simulink model "CMOS_Kernel_Memory_Sync"  (R2023b)
settings: Solver=VariableStepAuto  StartTime=0.0  StopTime=30000000  RelTol=1e-3
values from neighbouring files (symbols this model uses):
  AmountOfPixelsPerScanline = 400    [Kernel_Setup_Script.m]
  AmountOfRamBlocksScanlines = 5    [Kernel_Setup_Script.m]
  AmountOfRamBlocksScanlinesOffset = AmountOfRamBlocksScanlines - 1    (= 4)    [Kernel_Setup_Script.m]
  AmountOfScanlinePixels = 73700    [Kernel_Setup_Script.m]
  AmountOfScanlinePixelsOffset = AmountOfScanlinePixels - 1    (= 73699)    [Kernel_Setup_Script.m]
  AmountOfScanlines = 1100    [Kernel_Setup_Script.m]
  AmountOfScanlinesOffset = AmountOfScanlines - 1    (= 1099)    [Kernel_Setup_Script.m]
  AOPPK_Off = AmountOfPixelsPerScanline - 1    (= 399)    [Kernel_Setup_Script.m]
  AOPPS_Off = AmountOfPixelsPerScanline - 1    (= 399)    [Kernel_Setup_Script.m]
  FramePackOff_0 = FramePackOff_0 - ScanlineFifoCheck    [Kernel_Setup_Script.m]
  FramePackOff_1 = FramePackOff_1 - ScanlineFifoCheck    [Kernel_Setup_Script.m]
  FramePackOff_2 = FramePackOff_2 - ScanlineFifoCheck    [Kernel_Setup_Script.m]
  FramePackOff_3 = FramePackOff_3 - ScanlineFifoCheck    [Kernel_Setup_Script.m]
  FramePackOff_4 = FramePackOff_4 - ScanlineFifoCheck    [Kernel_Setup_Script.m]
  FramePackOff_5 = FramePackOff_5 - ScanlineFifoCheck    [Kernel_Setup_Script.m]
  KernelPackOff_0 = KernelPackOff_0 - KernelBitsPerRow    [Kernel_Setup_Script.m]
  KernelPackOff_1 = KernelPackOff_1 - KernelBitsPerRow    [Kernel_Setup_Script.m]
  KernelPackOff_2 = KernelPackOff_2 - KernelBitsPerRow    [Kernel_Setup_Script.m]
  KernelPackOff_3 = KernelPackOff_3 - KernelBitsPerRow    [Kernel_Setup_Script.m]
  Slice59DownTo48Top = (MsbOffset - (ScanlinePixelBitSizeController*1))    (= 59)    [Kernel_Setup_Script.m]
  Slice71DownTo60Top = (MsbOffset - (ScanlinePixelBitSizeController*0))    (= 71)    [Kernel_Setup_Script.m]
  TotalSectionsForFrames = AmountOfScanlines/AmountOfRamBlocksScanlines    (= 220)    [Kernel_Setup_Script.m]
  UltraRamRows = AmountOfPixelsPerScanline/ScanlineFifoCheck    [Kernel_Setup_Script.m]
  UltraRamRowsCeil = ceil(AmountOfPixelsPerScanline/ScanlineFifoCheck)    [Kernel_Setup_Script.m]
  UltraRamRowsKernel = AmountOfPixelsPerScanline/KernelBitsPerRow    (= 100)    [Kernel_Setup_Script.m]
  UltraRamRowsKernelCeil = ceil(AmountOfPixelsPerScanline/KernelBitsPerRow)    [Kernel_Setup_Script.m]
  UltraRamRowsMemorySectionOffset = UltraRamRowsCeil*AmountOfRamBlocksScanlines    [Kernel_Setup_Script.m]
  UltraRamRowsOffset = UltraRamRowsCeil - 1    [Kernel_Setup_Script.m]
undefined symbols (not defined in the file or in its folder): c, Down, sfvc784, Up, xck26
libraries: hdlBasic x4512, vmcUtilities x1
(part 1 of 39)
settings Model: Creator=Backm  LastModifiedBy=Backm

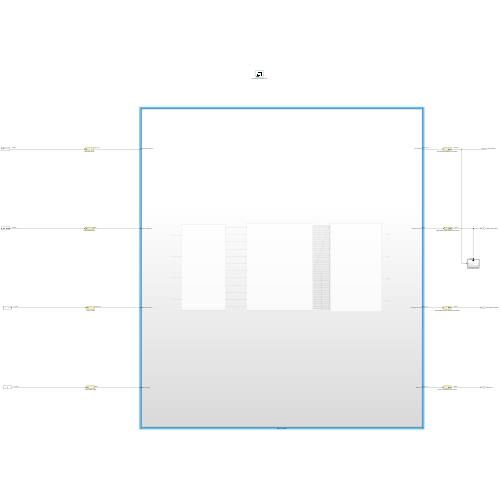
[thumbnail: Simulink's stored preview of the top-level diagram]
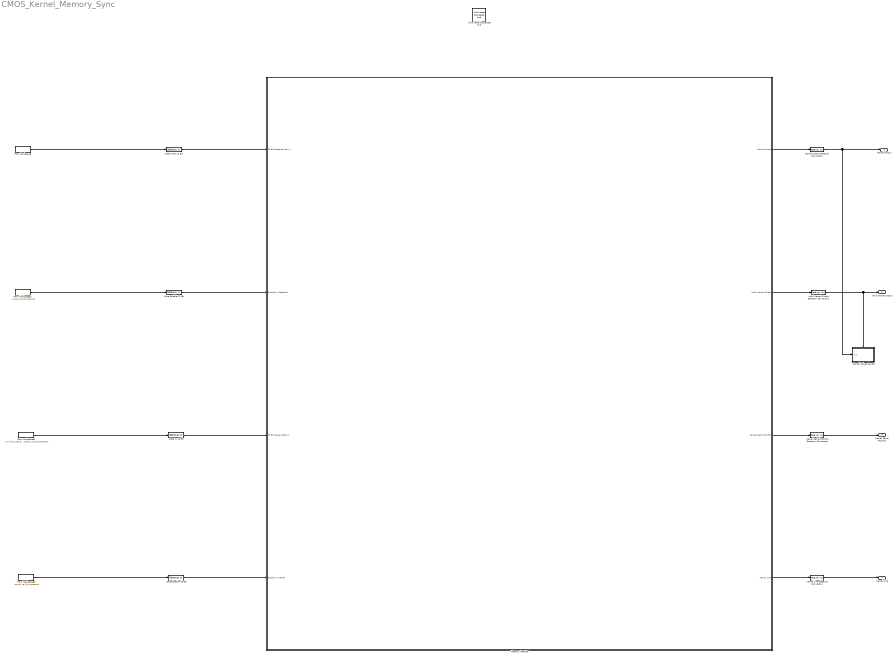
== system CMOS_Kernel_Memory_Sync ==
  Data Enable 18 Bit : hdlBasic/Gateway In  gui_display_data_type=Boolean  arith_type=Boolean  n_bits=18  bin_pt=0  preci_type=Single  exp_width=8  frac_width=24  rows=1  columns=1  quantization="Round  (unbiased: +/- Inf)"  overflow=Saturate  period=1  UseAsADC=off  ADCChannel='1'  interface=None  automatic_assignment=off  address_offset=hex2dec('00')  intf_name=''  intf_description=''  default_value=0  timing_constraint=None  locs_specified=off  LOCs={}  io_standard={}  inherit_from_input=off  hdl_port=on  XmcBlockStatus=1  maskContainerNames=group4  block_type=gatewayin  block_config=sysgen:gateway_in_config  block_width_w=590  block_height_w=620  block_width=640  block_height=850
  Data In 18 Bit : hdlBasic/Gateway In  gui_display_data_type=Fixed-point  arith_type=Unsigned  n_bits=18  bin_pt=0  preci_type=Single  exp_width=8  frac_width=24  rows=1  columns=1  quantization="Round  (unbiased: +/- Inf)"  overflow=Saturate  period=1  UseAsADC=off  ADCChannel='1'  interface=None  automatic_assignment=off  address_offset=hex2dec('00')  intf_name=''  intf_description=''  default_value=0  timing_constraint=None  locs_specified=off  LOCs={}  io_standard={}  inherit_from_input=off  hdl_port=on  XmcBlockStatus=1  maskContainerNames=group4  block_type=gatewayin  block_config=sysgen:gateway_in_config  block_width_w=590  block_height_w=620  block_width=640  block_height=850
  Data Input 12 Bit : hdlBasic/Gateway In  gui_display_data_type=Fixed-point  arith_type=Unsigned  n_bits=12  bin_pt=0  preci_type=Single  exp_width=8  frac_width=24  rows=1  columns=1  quantization="Round  (unbiased: +/- Inf)"  overflow=Saturate  period=1  UseAsADC=off  ADCChannel='1'  interface=None  automatic_assignment=off  address_offset=hex2dec('00')  intf_name=''  intf_description=''  default_value=0  timing_constraint=None  locs_specified=off  LOCs={}  io_standard={}  inherit_from_input=off  hdl_port=on  XmcBlockStatus=1  maskContainerNames=group4  block_type=gatewayin  block_config=sysgen:gateway_in_config  block_width_w=590  block_height_w=620  block_width=640  block_height=850
  From Workspace : FromWorkspace  VariableName=input_timeseries  Interpolate=off  OutputAfterFinalValue=Setting to zero
  From Workspace1 : FromWorkspace  VariableName=input_valid_timeseries  Interpolate=off  OutputAfterFinalValue=Setting to zero
  From Workspace2 : FromWorkspace  VariableName=auxillary_kernel_match_input_timeseries  Interpolate=off  OutputAfterFinalValue=Setting to zero
  From Workspace3 : FromWorkspace  VariableName=kernel_valid_timeseries  Interpolate=off  OutputAfterFinalValue=Setting to zero
  Kernel Line Gateway Conversion : hdlBasic/Gateway Out  inherit_from_input=off  hdl_port=on  rows=1  columns=1  UseAsDAC=off  DACChannel='1'  interface=None  automatic_assignment=on  address_offset=hex2dec('00')  intf_name=''  intf_description=''  timing_constraint=None  locs_specified=off  LOCs={}  io_standard={}  XmcBlockStatus=1  maskContainerNames=group4  block_type=gatewayout  block_config=sysgen:gateway_out_config  block_width_w=590  block_height_w=620  block_width=620  block_height=750
  Kernel Output Gateway Conversion : hdlBasic/Gateway Out  inherit_from_input=off  hdl_port=on  rows=1  columns=1  UseAsDAC=off  DACChannel='1'  interface=None  automatic_assignment=on  address_offset=hex2dec('00')  intf_name=''  intf_description=''  timing_constraint=None  locs_specified=off  LOCs={}  io_standard={}  XmcBlockStatus=1  maskContainerNames=group4  block_type=gatewayout  block_config=sysgen:gateway_out_config  block_width_w=590  block_height_w=620  block_width=620  block_height=750
  Kernel Serial Position Gateway Conversion : hdlBasic/Gateway Out  inherit_from_input=off  hdl_port=on  rows=1  columns=1  UseAsDAC=off  DACChannel='1'  interface=None  automatic_assignment=on  address_offset=hex2dec('00')  intf_name=''  intf_description=''  timing_constraint=None  locs_specified=off  LOCs={}  io_standard={}  XmcBlockStatus=1  maskContainerNames=group4  block_type=gatewayout  block_config=sysgen:gateway_out_config  block_width_w=590  block_height_w=620  block_width=620  block_height=750
  Kernel Values Saved : Subsystem
  Memory Handler : Subsystem
      settings: RTWMemSecFuncInitTerm=Inherit fRAM model  RTWMemSecFuncExecute=Inherit fRAM model  RTWMemSecDataConstants=Inherit fRAM model  RTWMemSecDataInternal=Inherit fRAM model  RTWMemSecDataParameters=Inherit fRAM model
  Valid Kernel Output Gateway Conversion : hdlBasic/Gateway Out  inherit_from_input=off  hdl_port=on  rows=1  columns=1  UseAsDAC=off  DACChannel='1'  interface=None  automatic_assignment=on  address_offset=hex2dec('00')  intf_name=''  intf_description=''  timing_constraint=None  locs_specified=off  LOCs={}  io_standard={}  XmcBlockStatus=1  maskContainerNames=group4  block_type=gatewayout  block_config=sysgen:gateway_out_config  block_width_w=590  block_height_w=620  block_width=620  block_height=750
  Vitis Model Composer Hub : vmcUtilities/Vitis Model Composer Hub  Tag=genX  CodeGeneration=off  SubsystemName=Frame Memory Controller  CompilationType=HDLCompilation  ExportTypeV2=IP Catalog  TargetDirectory=./netlist  exportDesign=off  analyzeDesign=off  validateDesignOnHw=off  ExportType=AI Engines  IpVendor=xilinx.com  IpLibrary=hls  IpVersion=1.0  IpHWLanguage=Verilog  AieCompilerOptions={}  AieSimulatorOptions={}  CreateTestbench=off  TestbenchStackSize=10  RunRtlSim=off  RunCSim=off  RunAieSim=off  AieSimTimeout=50000  RunAieSimProfiling=off  LaunchVitisAnalyzer=off  PlotOutput=off  RunX86Sim=off  X86SimTimeout=10  GenHwImage=off  GenLibadfXo=on  GenHwValidationCode=off  PlatformType=Not Specified  HwSystemType=Baremetal  HwValidationTarget=hw  ProjDevice=Kria KR260 Robotics Starter Kit SOM (xck26-sfvc784-2LV-c)  ProjDevicePart=xck26-sfvc784-2LV-c  SamplePeriod=-1  ClockFrequency=200  DataPathParallelism=1  xilinxfamily=zynquplus  part=xck26  speed=-2LV-c  package=sfvc784  directory=./netlist\ip\Frame_Memory_Controller\src  testbench=off  incr_netlist=off  synthesis_tool=Vivado  clock_wrapper=Clock Enables  dbl_ovrd=According to Block Masks  dcm_input_clock_period=10  sysclk_period=10  simulink_period=1/6  eval_field=0  LogFileName=''  NThreads=4
  Write Enable 12 Bit : hdlBasic/Gateway In  gui_display_data_type=Boolean  arith_type=Boolean  n_bits=16  bin_pt=14  preci_type=Single  exp_width=8  frac_width=24  rows=1  columns=1  quantization="Round  (unbiased: +/- Inf)"  overflow=Saturate  period=1  UseAsADC=off  ADCChannel='1'  interface=None  automatic_assignment=on  address_offset=hex2dec('00')  intf_name=''  intf_description=''  default_value=0  timing_constraint=None  locs_specified=off  LOCs={}  io_standard={}  inherit_from_input=off  hdl_port=on  XmcBlockStatus=1  maskContainerNames=group4  block_type=gatewayin  block_config=sysgen:gateway_in_config  block_width_w=590  block_height_w=620  block_width=640  block_height=850
  Kernel Output : Outport
  Valid Kernel Output : Outport  Port=2
  Kernel Serial Position : Outport  Port=3
  Kernel Line : Outport  Port=4
  wires:
  Kernel Line Gateway Conversion/1 -> Kernel Line/1
  Memory Handler/4(Kernel Line) -> Kernel Line Gateway Conversion/1
  Memory Handler/3(Kernel Serial Position) -> Kernel Serial Position Gateway Conversion/1
  Kernel Serial Position Gateway Conversion/1 -> Kernel Serial Position/1
  Memory Handler/2(Valid Kernel Output) -> Valid Kernel Output Gateway Conversion/1
  Valid Kernel Output Gateway Conversion/1 -> Valid Kernel Output/1, Kernel Values Saved/Enable
  Memory Handler/1(Kernel Output) -> Kernel Output Gateway Conversion/1
  Kernel Output Gateway Conversion/1 -> Kernel Output/1, Kernel Values Saved/1(In1)
  From Workspace/1 -> Data Input 12 Bit/1
  From Workspace1/1 -> Write Enable 12 Bit/1
  From Workspace2/1 -> Data In 18 Bit/1
  Data Enable 18 Bit/1 -> Memory Handler/4(Enable In Kernel)
  Data In 18 Bit/1 -> Memory Handler/3(18 Bit Kernel Data In)
  Write Enable 12 Bit/1 -> Memory Handler/2(Enable In Spectrual)
  Data Input 12 Bit/1 -> Memory Handler/1(12 Bit Spectrual Bin In)
  From Workspace3/1 -> Data Enable 18 Bit/1

== system CMOS_Kernel_Memory_Sync/Kernel Values Saved ==
  In1 : Inport
  Enable : EnablePort
  To Workspace : ToWorkspace  VariableName=simout_kernel_values_out  SampleTime=-1
      settings: Save2DSignal=2-D array (concatenate along first dimension)
  wires:
  In1/1 -> To Workspace/1

== system CMOS_Kernel_Memory_Sync/Memory Handler ==
  12 Bit Spectrual Bin In : Inport
  Enable In Spectrual : Inport  Port=2
  18 Bit Kernel Data In : Inport  Port=3
  Enable In Kernel : Inport  Port=4
  Data Slicer : Subsystem
      settings: RTWMemSecFuncInitTerm=Inherit fRAM model  RTWMemSecFuncExecute=Inherit fRAM model  RTWMemSecDataConstants=Inherit fRAM model  RTWMemSecDataInternal=Inherit fRAM model  RTWMemSecDataParameters=Inherit fRAM model
  Math : Subsystem
  Memory Manager : Subsystem
      settings: RTWMemSecFuncInitTerm=Inherit fRAM model  RTWMemSecFuncExecute=Inherit fRAM model  RTWMemSecDataConstants=Inherit fRAM model  RTWMemSecDataInternal=Inherit fRAM model  RTWMemSecDataParameters=Inherit fRAM model
  Kernel Output : Outport
  Valid Kernel Output : Outport  Port=2
  Kernel Serial Position : Outport  Port=3
  Kernel Line : Outport  Port=4
  wires:
  Memory Manager/11(Kernel RAM 4 Out1) -> Data Slicer/11(Kernel Data In RAM 4)
  12 Bit Spectrual Bin In/1 -> Memory Manager/1(12 Bit Spectrual Bin In)
  Memory Manager/2(Spectrual RAM 1 Out) -> Data Slicer/2(Data In RAM 1)
  Memory Manager/6(Spectrual Valid) -> Data Slicer/6(Frame Valid In)
  Memory Manager/4(Spectrual RAM 3 Out) -> Data Slicer/4(Data In RAM 3)
  Memory Manager/10(Kernel RAM 3 Out1) -> Data Slicer/10(Kernel Data In RAM 3)
  Memory Manager/3(Spectrual RAM 2 Out) -> Data Slicer/3(Data In RAM 2)
  Memory Manager/8(Kernel RAM 1 Out1) -> Data Slicer/8(Kernel Data In RAM 1)
  Memory Manager/9(Kernel RAM 2 Out1) -> Data Slicer/9(Kernel Data In RAM 2)
  Memory Manager/1(Spectrual RAM 0 Out) -> Data Slicer/1(Data In RAM 0)
  Memory Manager/7(Kernel RAM 0 Out1) -> Data Slicer/7(Kernel Data In RAM 0)
  Enable In Spectrual/1 -> Memory Manager/2(Enable In Spectrual)
  Memory Manager/12(" Kernel Valid") -> Data Slicer/12(Kernel Valid In)
  Memory Manager/5(Spectrual RAM 4 Out) -> Data Slicer/5(Data In RAM 4)
  Enable In Kernel/1 -> Memory Manager/4(Enable In Kernel)
  18 Bit Kernel Data In/1 -> Memory Manager/3(18 Bit Kernel Data In)
  Data Slicer/1(Frame Pixel 0 at Offset 0) -> Math/1(In Pixel 0 at Offset 0)
  Data Slicer/2(Frame Pixel 1 at Offset 0) -> Math/2(In Pixel 1 at Offset 0)
  Data Slicer/3(Frame Pixel 2 at Offset 0) -> Math/3(In Pixel 2 at Offset 0)
  Data Slicer/4(Frame Pixel 3 at Offset 0) -> Math/4(In Pixel 3 at Offset 0)
  Data Slicer/5(Frame Pixel 4 at Offset 0) -> Math/5(In Pixel 4 at Offset 0)
  Data Slicer/6(Frame Pixel 5 at Offset 0) -> Math/6(In Pixel 5 at Offset 0)
  Data Slicer/7(Frame Pixel 6 at Offset 0) -> Math/7(In Pixel 6 at Offset 0)
  Data Slicer/8(Frame Pixel 7 at Offset 0) -> Math/8(In Pixel 7 at Offset 0)
  Data Slicer/9(Frame Pixel 8 at Offset 0) -> Math/9(In Pixel 8 at Offset 0)
  Data Slicer/10(Frame Pixel 9 at Offset 0) -> Math/10(In Pixel 9 at Offset 0)
  Data Slicer/11(Frame Pixel 10 at Offset 0) -> Math/11(In Pixel 10 at Offset 0)
  Data Slicer/12(Frame Pixel 11 at Offset 0) -> Math/12(In Pixel 11 at Offset 0)
  Data Slicer/13(Frame Pixel 0 at Offset 1) -> Math/13(In Pixel 0 at Offset 1)
  Data Slicer/14(Frame Pixel 1 at Offset 1) -> Math/14(In Pixel 1 at Offset 1)
  Data Slicer/15(Frame Pixel 2 at Offset 1) -> Math/15(In Pixel 2 at Offset 1)
  Data Slicer/16(Frame Pixel 3 at Offset 1) -> Math/16(In Pixel 3 at Offset 1)
  Data Slicer/17(Frame Pixel 4 at Offset 1) -> Math/17(In Pixel 4 at Offset 1)
  Data Slicer/18(Frame Pixel 5 at Offset 1) -> Math/18(In Pixel 5 at Offset 1)
  Data Slicer/20(Frame Pixel 7 at Offset 1) -> Math/20(In Pixel 7 at Offset 1)
  Data Slicer/19(Frame Pixel 6 at Offset 1) -> Math/19(In Pixel 6 at Offset 1)
  Data Slicer/21(Frame Pixel 8 at Offset 1) -> Math/21(In Pixel 8 at Offset 1)
  Data Slicer/22(Frame Pixel 9 at Offset 1) -> Math/22(In Pixel 9 at Offset 1)
  Data Slicer/23(Frame Pixel 10 at Offset 1) -> Math/23(In Pixel 10 at Offset 1)
  Data Slicer/24(Frame Pixel 11 at Offset 1) -> Math/24(In Pixel 11 at Offset 1)
  Data Slicer/25(Frame Pixel 0 at Offset 2) -> Math/25(In Pixel 0 at Offset 2)
  Data Slicer/26(Frame Pixel 1 at Offset 2) -> Math/26(In Pixel 1 at Offset 2)
  Data Slicer/27(Frame Pixel 2 at Offset 2) -> Math/27(In Pixel 2 at Offset 2)
  Data Slicer/28(Frame Pixel 3 at Offset 2) -> Math/28(In Pixel 3 at Offset 2)
  Data Slicer/29(Frame Pixel 4 at Offset 2) -> Math/29(In Pixel 4 at Offset 2)
  Data Slicer/30(Frame Pixel 5 at Offset 2) -> Math/30(In Pixel 5 at Offset 2)
  Data Slicer/31(Frame Pixel 6 at Offset 2) -> Math/31(In Pixel 6 at Offset 2)
  Data Slicer/32(Frame Pixel 7 at Offset 2) -> Math/32(In Pixel 7 at Offset 2)
  Data Slicer/33(Frame Pixel 8 at Offset 2) -> Math/33(In Pixel 8 at Offset 2)
  Data Slicer/34(Frame Pixel 9 at Offset 2) -> Math/34(In Pixel 9 at Offset 2)
  Data Slicer/35(Frame Pixel 10 at Offset 2) -> Math/35(In Pixel 10 at Offset 2)
  Data Slicer/36(Frame Pixel 11 at Offset 2) -> Math/36(In Pixel 11 at Offset 2)
  Data Slicer/37(Frame Pixel 0 at Offset 3) -> Math/37(In Pixel 0 at Offset 3)
  Data Slicer/38(Frame Pixel 1 at Offset 3) -> Math/38(In Pixel 1 at Offset 3)
  Data Slicer/39(Frame Pixel 2 at Offset 3) -> Math/39(In Pixel 2 at Offset 3)
  Data Slicer/40(Frame Pixel 3 at Offset 3) -> Math/40(In Pixel 3 at Offset 3)
  Data Slicer/41(Frame Pixel 4 at Offset 3) -> Math/41(In Pixel 4 at Offset 3)
  Data Slicer/42(Frame Pixel 5 at Offset 3) -> Math/42(In Pixel 5 at Offset 3)
  Data Slicer/43(Frame Pixel 6 at Offset 3) -> Math/43(In Pixel 6 at Offset 3)
  Data Slicer/44(Frame Pixel 7 at Offset 3) -> Math/44(In Pixel 7 at Offset 3)
  Data Slicer/45(Frame Pixel 8 at Offset 3) -> Math/45(In Pixel 8 at Offset 3)
  Data Slicer/46(Frame Pixel 9 at Offset 3) -> Math/46(In Pixel 9 at Offset 3)
  Data Slicer/47(Frame Pixel 10 at Offset 3) -> Math/47(In Pixel 10 at Offset 3)
  Data Slicer/48(Frame Pixel 11 at Offset 3) -> Math/48(In Pixel 11 at Offset 3)
  Data Slicer/49(Frame Pixel 0 at Offset 4) -> Math/49(In Pixel 0 at Offset 4)
  Data Slicer/50(Frame Pixel 1 at Offset 4) -> Math/50(In Pixel 1 at Offset 4)
  Data Slicer/51(Frame Pixel 2 at Offset 4) -> Math/51(In Pixel 2 at Offset 4)
  Data Slicer/52(Frame Pixel 3 at Offset 4) -> Math/52(In Pixel 3 at Offset 4)
  Data Slicer/53(Frame Pixel 4 at Offset 4) -> Math/53(In Pixel 4 at Offset 4)
  Data Slicer/54(Frame Pixel 5 at Offset 4) -> Math/54(In Pixel 5 at Offset 4)
  Data Slicer/55(Frame Pixel 6 at Offset 4) -> Math/55(In Pixel 6 at Offset 4)
  Data Slicer/56(Frame Pixel 7 at Offset 4) -> Math/56(In Pixel 7 at Offset 4)
  Data Slicer/57(Frame Pixel 8 at Offset 4) -> Math/57(In Pixel 8 at Offset 4)
  Data Slicer/58(Frame Pixel 9 at Offset 4) -> Math/58(In Pixel 9 at Offset 4)
  Data Slicer/59(Frame Pixel 10 at Offset 4) -> Math/59(In Pixel 10 at Offset 4)
  Data Slicer/60(Frame Pixel 11 at Offset 4) -> Math/60(In Pixel 11 at Offset 4)
  Data Slicer/61(Weight 0 at Offset 0) -> Math/61(In Weight 0 at Offset 0)
  Data Slicer/62(Weight 1 at Offset 0) -> Math/62(In Weight 1 at Offset 0)
  Data Slicer/63(Weight 2 at Offset 0) -> Math/63(In Weight 2 at Offset 0)
  Data Slicer/64(Weight 3 at Offset 0) -> Math/64(In Weight 3 at Offset 0)
  Data Slicer/65(Weight 4 at Offset 0) -> Math/65(In Weight 4 at Offset 0)
  Data Slicer/66(Weight 5 at Offset 0) -> Math/66(In Weight 5 at Offset 0)
  Data Slicer/67(Weight 6 at Offset 0) -> Math/67(In Weight 6 at Offset 0)
  Data Slicer/68(Weight 7 at Offset 0) -> Math/68(In Weight 7 at Offset 0)
  Data Slicer/69(Weight 8 at Offset 0) -> Math/69(In Weight 8 at Offset 0)
  Data Slicer/70(Weight 9 at Offset 0) -> Math/70(In Weight 9 at Offset 0)
  Data Slicer/71(Weight 10 at Offset 0) -> Math/71(In Weight 10 at Offset 0)
  Data Slicer/72(Weight 11 at Offset 0) -> Math/72(In Weight 11 at Offset 0)
  Data Slicer/73(Weight 0 at Offset 1) -> Math/73(In Weight 0 at Offset 1)
  Data Slicer/74(Weight 1 at Offset 1) -> Math/74(In Weight 1 at Offset 1)
  Data Slicer/75(Weight 2 at Offset 1) -> Math/75(In Weight 2 at Offset 1)
  Data Slicer/76(Weight 3 at Offset 1) -> Math/76(In Weight 3 at Offset 1)
  Data Slicer/77(Weight 4 at Offset 1) -> Math/77(In Weight 4 at Offset 1)
  Data Slicer/78(Weight 5 at Offset 1) -> Math/78(In Weight 5 at Offset 1)
  Data Slicer/79(Weight 6 at Offset 1) -> Math/79(In Weight 6 at Offset 1)
  Data Slicer/80(Weight 7 at Offset 1) -> Math/80(In Weight 7 at Offset 1)
  Data Slicer/81(Weight 8 at Offset 1) -> Math/81(In Weight 8 at Offset 1)
  Data Slicer/82(Weight 9 at Offset 1) -> Math/82(In Weight 9 at Offset 1)
  Data Slicer/83(Weight 10 at Offset 1) -> Math/83(In Weight 10 at Offset 1)
  Data Slicer/84(Weight 11 at Offset 1) -> Math/84(In Weight 11 at Offset 1)
  Data Slicer/85(Weight 0 at Offset 2) -> Math/85(In Weight 0 at Offset 2)
  Data Slicer/86(Weight 1 at Offset 2) -> Math/86(In Weight 1 at Offset 2)
  Data Slicer/87(Weight 2 at Offset 2) -> Math/87(In Weight 2 at Offset 2)
  Data Slicer/88(Weight 3 at Offset 2) -> Math/88(In Weight 3 at Offset 2)
  Data Slicer/89(Weight 4 at Offset 2) -> Math/89(In Weight 4 at Offset 2)
  Data Slicer/90(Weight 5 at Offset 2) -> Math/90(In Weight 5 at Offset 2)
  Data Slicer/91(Weight 6 at Offset 2) -> Math/91(In Weight 6 at Offset 2)
  Data Slicer/92(Weight 7 at Offset 2) -> Math/92(In Weight 7 at Offset 2)
  Data Slicer/93(Weight 8 at Offset 2) -> Math/93(In Weight 8 at Offset 2)
  Data Slicer/94(Weight 9 at Offset 2) -> Math/94(In Weight 9 at Offset 2)
  Data Slicer/95(Weight 10 at Offset 2) -> Math/95(In Weight 10 at Offset 2)
  Data Slicer/96(Weight 11 at Offset 2) -> Math/96(In Weight 11 at Offset 2)
  Data Slicer/97(Weight 0 at Offset 3) -> Math/97(In Weight 0 at Offset 3)
  Data Slicer/98(Weight 1 at Offset 3) -> Math/98(In Weight 1 at Offset 3)
  Data Slicer/99(Weight 2 at Offset 3) -> Math/99(In Weight 2 at Offset 3)
  Data Slicer/100(Weight 3 at Offset 3) -> Math/100(In Weight 3 at Offset 3)
  Data Slicer/101(Weight 4 at Offset 3) -> Math/101(In Weight 4 at Offset 3)
  Data Slicer/102(Weight 5 at Offset 3) -> Math/102(In Weight 5 at Offset 3)
  Data Slicer/103(Weight 6 at Offset 3) -> Math/103(In Weight 6 at Offset 3)
  Data Slicer/104(Weight 7 at Offset 3) -> Math/104(In Weight 7 at Offset 3)
  Data Slicer/105(Weight 8 at Offset 3) -> Math/105(In Weight 8 at Offset 3)
  Data Slicer/106(Weight 9 at Offset 3) -> Math/106(In Weight 9 at Offset 3)
  Data Slicer/107(Weight 10 at Offset 3) -> Math/107(In Weight 10 at Offset 3)
  Data Slicer/108(Weight 11 at Offset 3) -> Math/108(In Weight 11 at Offset 3)
  Data Slicer/109(Weight 0 at Offset 4) -> Math/109(In Weight 0 at Offset 4)
  Data Slicer/110(Weight 1 at Offset 4) -> Math/110(In Weight 1 at Offset 4)
  Data Slicer/111(Weight 2 at Offset 4) -> Math/111(In Weight 2 at Offset 4)
  Data Slicer/112(Weight 3 at Offset 4) -> Math/112(In Weight 3 at Offset 4)
  Data Slicer/114(Weight 5 at Offset 4) -> Math/114(In Weight 5 at Offset 4)
  Data Slicer/113(Weight 4 at Offset 4) -> Math/113(In Weight 4 at Offset 4)
  Data Slicer/115(Weight 6 at Offset 4) -> Math/115(In Weight 6 at Offset 4)
  Data Slicer/116(Weight 7 at Offset 4) -> Math/116(In Weight 7 at Offset 4)
  Data Slicer/117(Weight 8 at Offset 4) -> Math/117(In Weight 8 at Offset 4)
  Data Slicer/118(Weight 9 at Offset 4) -> Math/118(In Weight 9 at Offset 4)
  Data Slicer/119(Weight 10 at Offset 4) -> Math/119(In Weight 10 at Offset 4)
  Data Slicer/120(Weight 11 at Offset 4) -> Math/120(In Weight 11 at Offset 4)
  Data Slicer/121(Valid Data) -> Math/121(Valid Data In)
  Math/4(Kernel Result Row Depth Position) -> Kernel Line/1
  Math/3(Kernel Result Array Position) -> Kernel Serial Position/1
  Math/2(Valid Kernel Output) -> Valid Kernel Output/1
  Math/1(Kernel Output) -> Kernel Output/1
